simulink model "simuTP2"  (R2020b)
settings: Solver=VariableStepAuto  StartTime=0.0  StopTime=10  RelTol=1e-3
undefined symbols (not defined in the file or in its folder): Fs
settings Model: Creator=Etudiants  LastModifiedBy=Etudiants

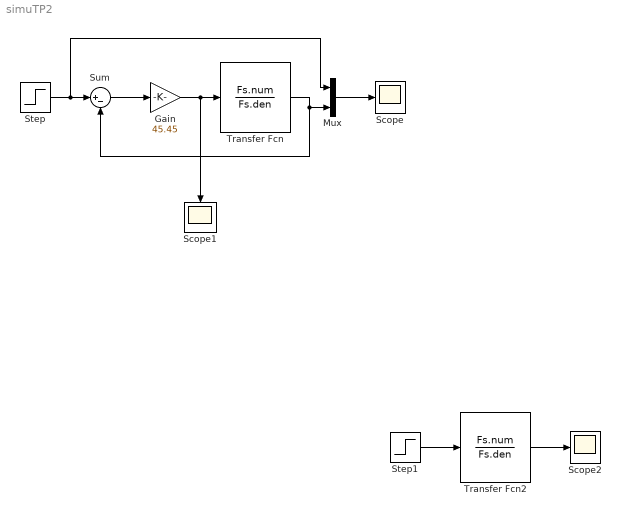
== system simuTP2 ==
  Gain : Gain  Gain=45.45
  Mux : Mux  Inputs=2
  Scope : Scope
  Scope1 : Scope
  Scope2 : Scope
  Step : Step  Time=0  SampleTime=0
  Step1 : Step  Time=0  After=2  SampleTime=0
  Sum : Sum  Inputs=|+-
  Transfer Fcn : TransferFcn  Numerator=Fs.num  Denominator=Fs.den
  Transfer Fcn2 : TransferFcn  Numerator=Fs.num  Denominator=Fs.den
  wires:
  Step/1 -> Sum/1, Mux/1
  Transfer Fcn/1 -> Mux/2, Sum/2
  Sum/1 -> Gain/1
  Gain/1 -> Scope1/1, Transfer Fcn/1
  Mux/1 -> Scope/1
  Step1/1 -> Transfer Fcn2/1
  Transfer Fcn2/1 -> Scope2/1
